simulink model "Solver"  (R2020a)
settings: Solver=FixedStepDiscrete  StartTime=0.0  StopTime=20  FixedStep=0.1  RelTol=1e-3
settings Model: OrderedModelArguments=off  Creator=ashok  LastModifiedBy=ashok
settings DataIOCC: ExternalInput=[t,u]

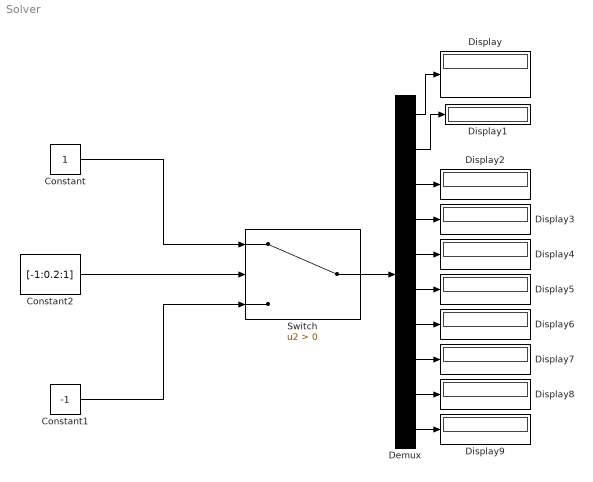
== system Solver ==
  Constant : Constant
  Constant1 : Constant  Value=-1
  Constant2 : Constant  Value=[-1:0.2:1]
  Demux : Demux  Outputs=10
  Display{,1..9} (10 alike) : Display
  Switch : Switch  Criteria=u2 > Threshold
  wires:
  Constant2/1 -> Switch/2
  Constant/1 -> Switch/1
  Constant1/1 -> Switch/3
  Switch/1 -> Demux/1
  Demux/1 -> Display/1
  Demux/2 -> Display1/1
  Demux/3 -> Display2/1
  Demux/4 -> Display3/1
  Demux/5 -> Display4/1
  Demux/6 -> Display5/1
  Demux/7 -> Display6/1
  Demux/8 -> Display7/1
  Demux/9 -> Display8/1
  Demux/10 -> Display9/1
